simulink model "six_02"  (R2021a)
settings: Solver=FixedStepDiscrete  StartTime=0.0  StopTime=50  FixedStep=0.1  RelTol=1e-3  EnableMultiTasking=on
settings Model: Creator=AlgoOy  LastModifiedBy=AlgoOy
settings SolverCC: AlgebraicLoopSolver=TrustRegion  AutoInsertRateTranBlk=on
settings DataIOCC: LimitDataPoints=on
settings OptimizationCC: LifeSpan=inf
settings DebuggingCC: AllowSymbolicDim=off  SFUnexpectedBacktrackingDiag=warning  SFNoUnconditionalDefaultTransitionDiag=warning  SFExecutionAtInitializationDiag=none  ArithmeticOperatorsInVariantConditions=warning
settings SFSimCC: SimUseLocalCustomCode=off  CustomCodeUndefinedFunction=UseInterfaceOnly
settings RTWCC: RTWUseLocalCustomCode=off
settings CodeAppCC: StateflowObjectComments=on
settings GRTTargetCC: TargetLangStandard=C89/C90 (ANSI)
settings ConfigComp: CovMetricSettings=dw  CovSaveCumulativeToWorkspaceVar=on  CovSaveSingleToWorkspaceVar=on  CovExternalEMLEnable=off

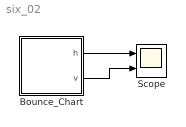
== system six_02 ==
  Bounce_Chart : Stateflow chart  TreatAsAtomicUnit=on
  Scope : Scope  NumInputPorts=2
  wires:
  Bounce_Chart/1(h) -> Scope/1
  Bounce_Chart/2(v) -> Scope/2

== stateflow chart six_02/Bounce_Chart ==
  state DOWN
    entry:
    t = 0;
    h = h0;
    v = v0;
    during:
    t = t + 0.01;
    v = 9.8 * t;
    h = h0 - 4.9 * t * t;
  state UP
    entry:
    t = 0;
    v = v0;
    during:
    t = t + 0.01;
    v = v0 + 9.8 * t;
    h = -v0 * t - 4.9 * t * t;
    h0 = h;
  (default) -> DOWN : {h0=2;v0 = 0;}
  DOWN -> UP : [h <= 0]{v0 = -0.8 * v}
  UP -> DOWN : [v >= 0]{v0 = 0}
  data: h output; v0 local; v output; t local; h0 local
